simulink library "carnot"  (R2018b)
settings: Solver=VariableStepAuto  StartTime=0.0  StopTime=10.0  RelTol=1e-3
undefined symbols (not defined in the file or in its folder): A, A_earth, acol, Acol, ActPower1, ActPower2, ActPower3, Ad, Ad0, Ar, Au, Au0, Azimuth_Angle, B, Bd, Bd0, Br, Bu, Bu0, C, c1, c2, c3, c33, c4, c5, c6, CarnotCallbacks_Density, CarnotCallbacks_Enthalpy, CarnotCallbacks_Enthalpy2Temperature, CarnotCallbacks_Entropy, CarnotCallbacks_Evaporation_Enthalpy, CarnotCallbacks_GlobalMessageLevel, CarnotCallbacks_Grashof, CarnotCallbacks_Heat_Capacity, CarnotCallbacks_Kinematic_Viscosity, CarnotCallbacks_PMV_PPD, CarnotCallbacks_Prandtl, CarnotCallbacks_Saturation_Property, CarnotCallbacks_Saturation_Temperature, CarnotCallbacks_Saturation_Value_Water, CarnotCallbacks_Specific_Volume, CarnotCallbacks_Thermal_Conductivity, CarnotCallbacks_Vapour_Content, CarnotCallbacks_Vapour_Pressure, Cd, Cdl, Cr, Cu, Davies, Dd, DE_TRY2010_04_averageYear, delta_grd, density, DiameterLastPiece, dl, DPConstant, DPLinear, DPQuadratic, Dr ... (+59)
libraries: $bdroot x429, simulink x36, simulink_extras x12
(part 7 of 22)

== system carnot/Control/Thermostat_Proportional ==
  note: u = (Tset - T + Play/2)
  note: y = operationPoint*(1 + 1/(proportianlRange-Play)) * u
  note: Limit output between 0...1
  T : Inport
  Tset : Inport  Port=2
  Backlash : Backlash  BacklashWidth=bl
  Gain1 : Gain  Gain=0.5
  Play : Constant  Value=bl
  Product : Product  Inputs=**/
  Saturation : Saturate  UpperLimit=1  LowerLimit=0
  Sensor : TransferFcn  Denominator=[ts 1]  mask{ts=ts}
      mask prompts: ts "First order hold for temperature sensor in s"
  Sum1 : Sum  Inputs=-++  SaturateOnIntegerOverflow=on  InputSameDT=on  OutDataTypeStr=Inherit: Same as first input
  Sum2 : Sum  Inputs=-+  SaturateOnIntegerOverflow=on  InputSameDT=on  OutDataTypeStr=Inherit: Same as first input
  Sum3 : Sum  Inputs=2  SaturateOnIntegerOverflow=on  InputSameDT=on  OutDataTypeStr=Inherit: Same as first input
  operationPosition : Constant  Value=op
  proportionalRange : Constant  Value=p
  pos : Outport
  wires:
  Sensor/1 -> Sum1/1
  Sum1/1 -> Backlash/1
  Backlash/1 -> Product/2  "u"
  Saturation/1 -> pos/1
  Sum3/1 -> Saturation/1
  T/1 -> Sensor/1
  Tset/1 -> Sum1/2
  Play/1 -> Sum2/1, Gain1/1
  Gain1/1 -> Sum1/3
  operationPosition/1 -> Sum3/1, Product/1
  proportionalRange/1 -> Sum2/2
  Sum2/1 -> Product/3
  Product/1 -> Sum3/2

== system carnot/Control/Window_Control ==
  Tamb : Inport
  Troom : Inport  Port=2
  Clock2 : Clock
  Data Type Conversion : DataTypeConversion
  FromMorning : simulink/Logic and Bit Operations/Compare To Constant  relop=>=  const=starttime  OutDataTypeStr=boolean
  J->kWh7 : Gain  Gain=1/3600  SaturateOnIntegerOverflow=on  OutDataTypeStr=Inherit: Same as input  ParamDataTypeStr=Inherit: Same as input
  Logical Operator : Logic  AllPortsSameDT=off  OutDataTypeStr=boolean
  Logical Operator1 : Logic  Inputs=3  AllPortsSameDT=off  OutDataTypeStr=boolean
  Math Function : Math  Operator=rem  SaturateOnIntegerOverflow=on
  MovingAverage : DiscreteFir  Coefficients=ones(1,floor(timeFIR))*(1/floor(timeFIR))  InitialStates=TaIni  SampleTime=3600  AccumDataTypeStr=Inherit: Same as product output  RndMeth=Nearest
  Product : Product  RndMeth=Zero
  RelayTroom : Relay  OnSwitchValue=Topen  OffSwitchValue=Tclose
  Rounding Function : Rounding
  Subtract : Sum  Inputs=+-
  Tamb_GT_Const : simulink/Logic and Bit Operations/Compare To Constant  relop=>=  const=TaTooCold  OutDataTypeStr=boolean
  TillEvening : simulink/Logic and Bit Operations/Compare To Constant  relop=<  const=stoptime  OutDataTypeStr=boolean
  Troom_GE_Tamb : simulink/Logic and Bit Operations/Compare To Constant  relop=>=  const=TrAboveTa  OutDataTypeStr=boolean
  const1 : Constant  Value=24*3600
  OpenWindow : Outport
  wires:
  Clock2/1 -> Math Function/1
  const1/1 -> Math Function/2
  Math Function/1 -> J->kWh7/1
  J->kWh7/1 -> Rounding Function/1
  Rounding Function/1 -> TillEvening/1, FromMorning/1  "hourOfTheDay"
  TillEvening/1 -> Logical Operator/1
  FromMorning/1 -> Logical Operator/2
  Tamb/1 -> Subtract/2, MovingAverage/1  "Tamb"
  Logical Operator/1 -> Logical Operator1/3  "daytime"
  Troom/1 -> Subtract/1, RelayTroom/1  "Troom"
  Subtract/1 -> Troom_GE_Tamb/1  "Tr-Ta"
  Troom_GE_Tamb/1 -> Logical Operator1/1  "Troom_GE_Tamb"
  Logical Operator1/1 -> Data Type Conversion/1
  Tamb_GT_Const/1 -> Logical Operator1/2  "Tamb_GT_Const"
  Data Type Conversion/1 -> Product/2
  Product/1 -> OpenWindow/1
  RelayTroom/1 -> Product/1  "TroomTooWarm"
  MovingAverage/1 -> Tamb_GT_Const/1  "TambAvg"

== system carnot/Hydraulics/Fan_Const ==
  THB_Air : Inport
  Ctrl : Inport  Port=2
  Pump_Const : $bdroot/Hydraulics/Pump_Const  mdotmax=Vdotmax/3600*density(Tini,p0,2,0)  dia=dia  p0=p0  fluid_id=Air  mix=mix  mix2=0  mix3=0  UA=UA  mcp=mcp  Tini=Tini  e0=e0  e1=e1  e2=e2
  THB : Outport
  FanDat : Outport  Port=2
  wires:
  Pump_Const/2 -> FanDat/1
  Pump_Const/1 -> THB/1
  Ctrl/1 -> Pump_Const/2  "ControlSetpoint"
  THB_Air/1 -> Pump_Const/1

== system carnot/Hydraulics/Flow_Diverter ==
  THB : Inport
  fdiv : Inport  Port=2
  Bus Assignment : BusAssignment  AssignedSignals=ID,MassFlow,DPConstant,DPLinear,DPQuadratic
  Bus Assignment1 : BusAssignment  AssignedSignals=ID,MassFlow,DPConstant,DPLinear,DPQuadratic
  Bus Selector10 : BusSelector  OutputSignals=MassFlow,DPConstant,DPLinear,DPQuadratic  OutputAsBus=on
  Bus Selector : BusSelector  OutputSignals=MassFlow
  Bus Selector4 : BusSelector  OutputSignals=ID
  Dot Product : DotProduct  InputSameDT=on  OutDataTypeStr=Inherit: Inherit via internal rule
  Saturation : Saturate  UpperLimit=1  LowerLimit=0
  Sum : Sum  Inputs=-+  SaturateOnIntegerOverflow=on  InputSameDT=on  OutDataTypeStr=Inherit: Same as first input
  const{,1..2,4..6} (6 alike) : Constant  Value=0
  increase_ID : Subsystem
  THB1 : Outport
  THB2 : Outport  Port=2
  clq : Outport  Port=3
  wires:
  Bus Selector10/1 -> clq/1
  Bus Assignment1/1 -> THB2/1
  Bus Assignment/1 -> THB1/1
  const4/1 -> Bus Assignment/4  "DPConstant"
  const5/1 -> Bus Assignment/5  "DPLinear"
  const6/1 -> Bus Assignment/6  "DPQuadratic"
  increase_ID/1(Out1) -> Bus Assignment1/2, Bus Assignment/2  "ID"
  Bus Selector4/1 -> increase_ID/1(In1)  "<ID>"
  Dot Product/1 -> Bus Assignment/3, Sum/1  "MassFlow"
  fdiv/1 -> Saturation/1
  THB/1 -> Bus Assignment1/1, Bus Selector10/1, Bus Selector4/1, Bus Assignment/1, Bus Selector/1
  const/1 -> Bus Assignment1/4  "DPConstant"
  Bus Selector/1 -> Sum/2, Dot Product/1  "<MassFlow>"
  Sum/1 -> Bus Assignment1/3  "MassFlow"
  Saturation/1 -> Dot Product/2
  const1/1 -> Bus Assignment1/5  "DPLinear"
  const2/1 -> Bus Assignment1/6  "DPQuadratic"

== system carnot/Hydraulics/Flow_Mixer ==
  THB1 : Inport
  THB2 : Inport  Port=2
  clq : Inport  Port=3
  Calculate_fdiv : Subsystem
  Flow_Mixer_basic : $bdroot/Basic/Hydraulics/Flow_Mixer_basic
  THB : Outport
  fdiv : Outport  Port=2
  wires:
  clq/1 -> Flow_Mixer_basic/3
  Calculate_fdiv/1(f_div) -> fdiv/1
  THB1/1 -> Flow_Mixer_basic/1
  THB2/1 -> Flow_Mixer_basic/2
  Flow_Mixer_basic/1 -> THB/1
  Flow_Mixer_basic/2 -> Calculate_fdiv/1(ID_1)
  Flow_Mixer_basic/3 -> Calculate_fdiv/2(ID_2)
  Flow_Mixer_basic/4 -> Calculate_fdiv/3(fdiv)

== system carnot/Hydraulics/Flow_Mixer_Thermostatic ==
  THBhot : Inport
  THBcold : Inport  Port=2
  clq : Inport  Port=3
  Tset : Inport  Port=4
  Bus Selector : BusSelector  OutputSignals=Temperature
  Flow_Mixer_basic : $bdroot/Basic/Hydraulics/Flow_Mixer_basic
  Icontrol_fdiv : Subsystem
  Terminator : Terminator
  THB : Outport
  fdiv : Outport  Port=2
  wires:
  Bus Selector/1 -> Icontrol_fdiv/3(Twarm)  "<Temperature>"
  Flow_Mixer_basic/4 -> Terminator/1
  Tset/1 -> Icontrol_fdiv/4(Tset)
  Flow_Mixer_basic/3 -> Icontrol_fdiv/2(ID_2)
  Flow_Mixer_basic/2 -> Icontrol_fdiv/1(ID_1)
  Flow_Mixer_basic/1 -> Bus Selector/1, THB/1
  clq/1 -> Flow_Mixer_basic/3
  THBcold/1 -> Flow_Mixer_basic/2
  THBhot/1 -> Flow_Mixer_basic/1
  Icontrol_fdiv/1(f_div) -> fdiv/1

== system carnot/Hydraulics/Mixing_Valve ==
  THB_A : Inport
  THB_B : Inport  Port=2
  clq : Inport  Port=3
  Ctrl : Inport  Port=4
  Bus Creator : BusCreator  Inputs=2
  Calculate_fdiv : Subsystem
  Fcn : Fcn  Expr=1-u
  Flow_Mixer_basic : $bdroot/Basic/Hydraulics/Flow_Mixer_basic
  Valve_A : $bdroot/Hydraulics/Valve  vtyp=equal percentage  psi_0=psi_0  kvs=kvs  dt_V=dt_V
  Valve_B : $bdroot/Hydraulics/Valve  vtyp=linear  psi_0=psi_0  kvs=kvs  dt_V=dt_V
  THB_AB : Outport
  fdiv : Outport  Port=2
  pos : Outport  Port=3
  wires:
  Flow_Mixer_basic/4 -> Calculate_fdiv/3(fdiv)
  Flow_Mixer_basic/3 -> Calculate_fdiv/2(ID_2)
  Flow_Mixer_basic/2 -> Calculate_fdiv/1(ID_1)
  Flow_Mixer_basic/1 -> THB_AB/1
  THB_A/1 -> Valve_A/1
  Calculate_fdiv/1(f_div) -> fdiv/1
  clq/1 -> Flow_Mixer_basic/3
  Valve_A/1 -> Flow_Mixer_basic/1
  THB_B/1 -> Valve_B/1
  Ctrl/1 -> Fcn/1, Valve_A/2
  Valve_B/1 -> Flow_Mixer_basic/2
  Bus Creator/1 -> pos/1
  Valve_A/2 -> Bus Creator/1  "pos_A"
  Valve_B/2 -> Bus Creator/2  "pos_B"
  Fcn/1 -> Valve_B/2

== system carnot/Hydraulics/Pipe ==
  Tamb : Inport
  THBin : Inport  Port=2
  Constant : Constant  Value=hgt
  Pipe_basic : $bdroot/Basic/Thermal_Models/Pipe_basic  vol=pi*(dia/2)^2*len  L=len  uloss=uloss  effcond=cond  cwall=cwall  t0=t0  nodes=nodes
  Pressure_Drop_Fix : $bdroot/Basic/Pressure_Drop/Pressure_Drop_Fix  con=0  lin=lin  qua=qua
  Pressure_Drop_changeD : $bdroot/Basic/Pressure_Drop/Pressure_Drop_changeD  dia=dia
  Pressure_Drop_staticHeight : $bdroot/Basic/Pressure_Drop/Pressure_Drop_staticHeight
  THB : Outport
  wires:
  Pipe_basic/2 -> Pressure_Drop_staticHeight/2
  Pipe_basic/1 -> Pressure_Drop_staticHeight/1
  Tamb/1 -> Pipe_basic/1
  THBin/1 -> Pipe_basic/2
  Constant/1 -> Pressure_Drop_staticHeight/3
  Pressure_Drop_staticHeight/1 -> Pressure_Drop_Fix/1
  Pressure_Drop_Fix/1 -> Pressure_Drop_changeD/1
  Pressure_Drop_changeD/1 -> THB/1

== system carnot/Hydraulics/Pipe_BiFlow ==
  note: discharging pipe connection
  note: charging pipe connection
  Tamb : Inport
  THB_1_in : Inport  Port=2
  THB_2_in : Inport  Port=3
  Constant_THB : $bdroot/Source/Simple/Constant_THB  t=20  mdot=0  p=1e5  mID=No Pressure Drop  fluid=Water  mix=0  mix2=0  mix3=0  dia=0.02  hgt=0
  CreateSdat : $bdroot/Basic/Thermal_Models/CreateSdat  volume=volume  stgtype=stgtype
  Pipe_Connection_1 : $bdroot/Storage/Thermal/Storage_Ports/Pipe_Connection  h_in=pipe1inlet  h_out=pipe1outlet  hgt=hgt  dpipe=pipe1dia  dstg=dia  height=-1273.2395  nodes=nodes
  Pipe_Connection_2 : $bdroot/Storage/Thermal/Storage_Ports/Pipe_Connection  h_in=pipe2inlet  h_out=pipe2outlet  hgt=hgt  dpipe=pipe2dia  dstg=dia  height=1273.2395  nodes=nodes
  select_T : Selector  InputPortWidth=nodes  IndexOptions=Index vector (dialog)  Indices=[1 2 3 4 5 6 7 8 9 10]  OutputSizes=1
  sfun_storageTnodes : $bdroot/Basic/Thermal_Models/sfun_storageTnodes  uloss=uwall  ubot=ubot  utop=utop  cond=axcond  volume=volume  dia=dia  standing=standing cylinder  tini=tini  nodes=nodes  nconnect=2  elimthermocline=0  condinvtc=0
  Sdat : Outport
  THB_1_out : Outport  Port=2
  THB_2_out : Outport  Port=3
  wires:
  Constant_THB/1 -> CreateSdat/15, CreateSdat/8, CreateSdat/9, CreateSdat/10, CreateSdat/11, CreateSdat/12, CreateSdat/13, CreateSdat/14
  Pipe_Connection_1/1 -> sfun_storageTnodes/2
  Pipe_Connection_1/2 -> THB_1_out/1, CreateSdat/5  "THBoutPipe1"
  THB_1_in/1 -> Pipe_Connection_1/2, CreateSdat/4  "THBinPipe1"
  CreateSdat/1 -> Sdat/1
  sfun_storageTnodes/2 -> select_T/1, Pipe_Connection_1/1, Pipe_Connection_2/1  "Tnodes"
  select_T/1 -> CreateSdat/3  "Tnodes"
  Tamb/1 -> CreateSdat/1, sfun_storageTnodes/1  "Tamb"
  THB_2_in/1 -> CreateSdat/6, Pipe_Connection_2/2  "THBinPipe2"
  Pipe_Connection_2/1 -> sfun_storageTnodes/3
  Pipe_Connection_2/2 -> THB_2_out/1, CreateSdat/7  "THBoutPipe2"
  sfun_storageTnodes/1 -> CreateSdat/2  "Energy"

== system carnot/Hydraulics/Pipe_Geometry ==
  Tamb : Inport
  THBin : Inport  Port=2
  Constant : Constant  Value=hgt
  Pipe_basic : $bdroot/Basic/Thermal_Models/Pipe_basic  vol=pi*(dia/2)^2*len  L=len  uloss=uloss  effcond=cond  cwall=cwall  t0=t0  nodes=nodes
  Pressure_Drop_PipeTheory : $bdroot/Basic/Pressure_Drop/Pressure_Drop_PipeTheory  dia=dia  len=len  rough=rough  nbend=nbend
  Pressure_Drop_changeD : $bdroot/Basic/Pressure_Drop/Pressure_Drop_changeD  dia=dia
  Pressure_Drop_staticHeight : $bdroot/Basic/Pressure_Drop/Pressure_Drop_staticHeight
  THB : Outport
  wires:
  Pressure_Drop_PipeTheory/1 -> Pressure_Drop_changeD/1
  Pressure_Drop_staticHeight/1 -> Pressure_Drop_PipeTheory/2
  Pressure_Drop_changeD/1 -> THB/1
  Constant/1 -> Pressure_Drop_staticHeight/3
  Pipe_basic/2 -> Pressure_Drop_staticHeight/2
  Pipe_basic/1 -> Pressure_Drop_PipeTheory/1, Pressure_Drop_staticHeight/1
  THBin/1 -> Pipe_basic/2
  Tamb/1 -> Pipe_basic/1

== system carnot/Hydraulics/Pipe_Isolation ==
  Tamb : Inport
  THBin : Inport  Port=2
  Constant : Constant  Value=hgt
  Pipe_basic : $bdroot/Basic/Thermal_Models/Pipe_basic  vol=pi*(dia/2)^2*len  L=len  uloss=uloss  effcond=cond  cwall=cwall  t0=t0  nodes=nodes
  Pressure_Drop_Fix : $bdroot/Basic/Pressure_Drop/Pressure_Drop_Fix  con=0  lin=lin  qua=qua
  Pressure_Drop_changeD : $bdroot/Basic/Pressure_Drop/Pressure_Drop_changeD  dia=dia
  Pressure_Drop_staticHeight : $bdroot/Basic/Pressure_Drop/Pressure_Drop_staticHeight
  THB : Outport
  wires:
  Pipe_basic/2 -> Pressure_Drop_staticHeight/2
  Pipe_basic/1 -> Pressure_Drop_staticHeight/1
  Pressure_Drop_changeD/1 -> THB/1
  Pressure_Drop_Fix/1 -> Pressure_Drop_changeD/1
  Pressure_Drop_staticHeight/1 -> Pressure_Drop_Fix/1
  Constant/1 -> Pressure_Drop_staticHeight/3
  THBin/1 -> Pipe_basic/2
  Tamb/1 -> Pipe_basic/1

== system carnot/Hydraulics/Pump_Additional ==
  note: Correct the negative pressuredrop.
      | Pump head increases the pressure.
  note: Control signal equal to zero switches
      | to negative ID -> no massflow in the
      | pump (and no pressure drop calculations
      | necessary in the components of the
      | hydraulic loop)
  note: Node for thermal losses and to break
      | the algebraic loop in the temperature
  THBin : Inport
  Ctrl : Inport  Port=2
  Abs : Abs
  Bus Assignment : BusAssignment  AssignedSignals=ID,Temperature,Pressure,DiameterLastPiece,DPConstant,DPLinear,DPQuadratic
  Bus Creator : BusCreator  Inputs=5
  Bus Selector1 : BusSelector  OutputSignals=ID
  Bus Selector2 : BusSelector  OutputSignals=MassFlow
  Bus Selector5 : BusSelector  OutputSignals=MassFlow,Pressure
  Demux : Demux  Outputs=3
  ElectricConsumptionPump : $bdroot/Basic/Hydraulics/ElectricConsumptionPump  e0=e0  e1=e1  e2=e2
  Gain{,1..3} (4 alike) : Gain  Gain=-1
  Pressuredrop : $bdroot/Basic/Pressure_Drop/Pressuredrop
  PumpHead : Gain  Gain=a0
  PumpLinear : Constant  Value=a1
  PumpQuadratic : Constant  Value=a2
  Saturation : Saturate  UpperLimit=1  LowerLimit=0
  Switch3 : Switch  Criteria=u2 > Threshold  SaturateOnIntegerOverflow=on  InputSameDT=on
  ThermalNodeTHB : $bdroot/Basic/Thermal_Models/ThermalNodeTHB  UA=UA  mcp=mcp  Tini=Tini
  dia : Constant  Value=dia
  gain1 : Gain  Gain=-1  SaturateOnIntegerOverflow=on  OutDataTypeStr=Inherit: Same as input  ParamDataTypeStr=Inherit: Same as input
  select_clq : Subsystem
  THB : Outport
  Pdat : Outport  Port=2
  wires:
  Saturation/1 -> Switch3/2, PumpHead/1, Bus Creator/4, ElectricConsumptionPump/2  "ControlActual"
  Gain3/1 -> Bus Creator/3  "PumpHead"
  Pressuredrop/1 -> Bus Assignment/4
  Pressuredrop/2 -> Demux/1  "clq_out"
  Pressuredrop/3 -> Gain3/1
  Bus Assignment/1 -> THB/1, Bus Creator/1  "THB"
  Bus Selector2/1 -> ElectricConsumptionPump/1  "<MassFlow>"
  Bus Creator/1 -> Pdat/1  "Pdat"
  ElectricConsumptionPump/1 -> Bus Creator/2  "PowerElectric"
  Ctrl/1 -> Saturation/1, Bus Creator/5  "ControlSetpoint"
  Bus Selector1/1 -> Switch3/1, Abs/1  "<ID>"
  Abs/1 -> gain1/1
  gain1/1 -> Switch3/3
  Switch3/1 -> Bus Assignment/2  "ID"
  Bus Selector5/1 -> Pressuredrop/1  "<MassFlow>"
  dia/1 -> Bus Assignment/5
  THBin/1 -> select_clq/1(THB), Bus Selector2/1, Bus Selector5/1, Bus Selector1/1, ThermalNodeTHB/1, Bus Assignment/1
  PumpHead/1 -> Gain/1
  PumpLinear/1 -> Gain1/1
  PumpQuadratic/1 -> Gain2/1
  Demux/1 -> Bus Assignment/6
  Demux/2 -> Bus Assignment/7
  Demux/3 -> Bus Assignment/8
  ThermalNodeTHB/1 -> Bus Assignment/3
  select_clq/1(clq) -> Pressuredrop/3
  Bus Selector5/2 -> Pressuredrop/2  "<Pressure>"
  Gain/1 -> Pressuredrop/4
  Gain1/1 -> Pressuredrop/5
  Gain2/1 -> Pressuredrop/6

== system carnot/Hydraulics/Pump_Const ==
  THBin : Inport
  Ctrl : Inport  Port=2
  Bus Assignment : BusAssignment  AssignedSignals=Temperature
  Bus Creator : BusCreator  Inputs=5
  Bus Selector : BusSelector  OutputSignals=MassFlow
  ElectricConsumptionPump : $bdroot/Basic/Hydraulics/ElectricConsumptionPump  e0=e0  e1=e1  e2=e2
  PumpHead : Constant  Value=0
  Pump_basic : $bdroot/Hydraulics/Pump_basic  mdotmax=mdotmax  fluid_id=Water  mix=mix  mix2=mix2  mix3=mix3  p0=p0  dia=dia  ID=No Pressure Drop  hgt=0
  Saturation : Saturate  UpperLimit=1  LowerLimit=0
  ThermalNodeTHB : $bdroot/Basic/Thermal_Models/ThermalNodeTHB  UA=UA  mcp=mcp  Tini=Tini
  THB : Outport
  Pdat : Outport  Port=2
  wires:
  ThermalNodeTHB/1 -> Bus Assignment/2
  Saturation/1 -> Pump_basic/2, ElectricConsumptionPump/2, Bus Creator/4  "ControlActual"
  ElectricConsumptionPump/1 -> Bus Creator/2  "PowerElectric"
  Bus Creator/1 -> Pdat/1  "Pdat"
  Bus Assignment/1 -> THB/1, Bus Creator/1  "THB"
  PumpHead/1 -> Bus Creator/3  "PumpHead"
  Pump_basic/1 -> ThermalNodeTHB/1, Bus Selector/1, Bus Assignment/1
  THBin/1 -> Pump_basic/1
  Ctrl/1 -> Bus Creator/5, Saturation/1  "ControlSetpoint"
  Bus Selector/1 -> ElectricConsumptionPump/1  "<MassFlow>"

== system carnot/Hydraulics/Pump_Main ==
  note: Control signal equal to zero switches
      | to negative ID -> no massflow in the
      | pump (and no pressure drop calculations
      | necessary in the components of the
      | hydraulic loop)
  note: solve quadratic equation
      | DPCOnstant + DPLinear * mdot + DPQadraic * mdot^2
      | = a0 + a1 * mdot + a2 * mdot^2
  note: Transfer function to
      | break algebraic loop
      | in the massflow
  note: Node for thermal losses and to break
      | the algebraic loop in the temperature
  THBin : Inport
  Ctrl : Inport  Port=2
  Bus Assignment : BusAssignment  AssignedSignals=ID,Temperature,MassFlow,Pressure
  Bus Creator : BusCreator  Inputs=5
  Bus Selector : BusSelector  OutputSignals=ID,DPConstant,DPLinear,DPQuadratic
  ElectricConsumptionPump : $bdroot/Basic/Hydraulics/ElectricConsumptionPump  e0=e0  e1=e1  e2=e2
  Gain{1..4} (4 alike) : Gain  Gain=-1
  Ground : Ground
  ID : Constant  Value=ID  mask{IDpreset=pressure drop}
      mask prompts: IDpreset "Calculation"
      mask init:
      | ID = IDpreset*10000 + 1;
      mask TypeOptions IDpreset: pressure drop | pressure drop and pressure head
  Mux2 : Mux  Inputs=7
  Pressure : Constant  Value=p0
  Pressuredrop : $bdroot/Basic/Pressure_Drop/Pressuredrop
  PumpHead : Gain  Gain=a0
  PumpLinear : Constant  Value=a1
  PumpQuadratic : Constant  Value=a2
  S-Function : S-Function  FunctionName=pump  SFunctionDeploymentMode=off  EnableBusSupport=off
  Saturation : Saturate  UpperLimit=1  LowerLimit=0
  Switch1 : Switch  Criteria=u2 > Threshold  SaturateOnIntegerOverflow=on  InputSameDT=on
  Switch3 : Switch  Criteria=u2 > Threshold  SaturateOnIntegerOverflow=on  InputSameDT=on
  Terminator : Terminator
  ThermalNodeTHB : $bdroot/Basic/Thermal_Models/ThermalNodeTHB  UA=UA  mcp=mcp  Tini=Tini
  Transfer Fcn : TransferFcn  Denominator=[t1 1]  mask{t1=t1}
      mask prompts: t1 "Time constant of PT1 transfer function for massflow in s"
  basic_THB : $bdroot/Basic/Hydraulics/basic_THB  t=20  mdot=0  p=p0  ID=No Pressure Drop  fluid=Water  mix=mix  mix2=mix2  mix3=mix3  dia=dia  hgt=0
  const5 : Constant  Value=0
  gain1 : Gain  Gain=-1  SaturateOnIntegerOverflow=on  OutDataTypeStr=Inherit: Same as input  ParamDataTypeStr=Inherit: Same as input
  THB : Outport
  Pdat : Outport  Port=2
  wires:
  Gain4/1 -> Bus Creator/3  "PumpHead"
  Gain2/1 -> Pressuredrop/6
  Gain1/1 -> Pressuredrop/5
  Gain3/1 -> Pressuredrop/4
  Saturation/1 -> Bus Creator/4, ElectricConsumptionPump/2, PumpHead/1, Switch3/2  "ControlActual"
  Pressuredrop/2 -> Terminator/1
  Ground/1 -> Pressuredrop/3
  Pressuredrop/1 -> Bus Assignment/5
  Pressure/1 -> Pressuredrop/2
  Bus Selector/4 -> Mux2/4  "<DPQuadratic>"
  Bus Selector/3 -> Mux2/3  "<DPLinear>"
  Bus Selector/2 -> Mux2/2  "<DPConstant>"
  ThermalNodeTHB/1 -> Bus Assignment/3
  Switch3/1 -> Bus Assignment/2
  Bus Assignment/1 -> Bus Creator/1, THB/1  "THB"
  basic_THB/1 -> Bus Assignment/1
  const5/1 -> Switch1/3
  Transfer Fcn/1 -> Switch1/1, Pressuredrop/1
  gain1/1 -> Switch3/3
  ID/1 -> gain1/1, Switch3/1
  Ctrl/1 -> Bus Creator/5, Saturation/1  "ControlSetpoint"
  PumpHead/1 -> Mux2/5, Gain3/1
  PumpQuadratic/1 -> Mux2/7, Gain2/1
  PumpLinear/1 -> Mux2/6, Gain1/1
  S-Function/1 -> Transfer Fcn/1
  Mux2/1 -> S-Function/1
  Switch1/1 -> ElectricConsumptionPump/1, Bus Assignment/4  "MassFlow"
  Bus Selector/1 -> Mux2/1, Switch1/2  "<ID>"
  Pressuredrop/3 -> Gain4/1
  THBin/1 -> ThermalNodeTHB/1, Bus Selector/1
  Bus Creator/1 -> Pdat/1  "Pdat"
  ElectricConsumptionPump/1 -> Bus Creator/2  "PowerElectric"

== system carnot/Hydraulics/Pump_basic ==
  THBin : Inport
  Ctrl : Inport  Port=2
  Bus Assignment : BusAssignment  AssignedSignals=Temperature,MassFlow
  Bus Selector : BusSelector  OutputSignals=Temperature
  IC : InitialCondition  Value=20
  basic_THB : $bdroot/Basic/Hydraulics/basic_THB  t=20  mdot=0  p=p0  ID=No Pressure Drop  fluid=Water  mix=mix  mix2=mix2  mix3=mix3  dia=dia  hgt=hgt
  mdot : Gain  Gain=mdotmax  SaturateOnIntegerOverflow=on  OutDataTypeStr=Inherit: Same as input  ParamDataTypeStr=Inherit: Same as input
  THB : Outport
  wires:
  IC/1 -> Bus Assignment/2  "Temperature"
  mdot/1 -> Bus Assignment/3  "MassFlow"
  Ctrl/1 -> mdot/1
  THBin/1 -> Bus Selector/1
  Bus Selector/1 -> IC/1  "<Temperature>"
  basic_THB/1 -> Bus Assignment/1
  Bus Assignment/1 -> THB/1

== system carnot/Hydraulics/Thermosyphon ==
  note: Transfer function to
      | break algebraic loop
      | in the massflow
  THBin : Inport
  Bus Assignment : BusAssignment  AssignedSignals=Temperature,MassFlow
  Bus Selector1 : BusSelector  OutputSignals=DPConstant,DPLinear,DPQuadratic  OutputAsBus=on
  Bus Selector2 : BusSelector  OutputSignals=ID
  Bus Selector3 : BusSelector  OutputSignals=GeodeticHeight  OutputAsBus=on
  Bus Selector4 : BusSelector  OutputSignals=Temperature  OutputAsBus=on
  Check difference in height : simulink/Model Verification/Check  Static Range  Description=-0.001 <= u <= 0.001  max=0.001  max_included=on  min=-0.001  min_included=on  enabled=on  stopWhenAssertionFail=on  export=off  icon=graphic
      settings: SourceProductName=Simulink  SourceProductBaseCode=SL
  Mux2 : Mux  Inputs=5
  S-Function : S-Function  FunctionName=pump  SFunctionDeploymentMode=off  EnableBusSupport=off
  Switch1 : Switch  Criteria=u2 > Threshold  SaturateOnIntegerOverflow=on  InputSameDT=on
  Transfer Fcn : $bdroot/Hydraulics/Pump_Main/Transfer Fcn  t1=t1
  basic_THB : $bdroot/Basic/Hydraulics/basic_THB  t=20  mdot=0  p=p0  ID=Full Pressure Drop with Static Height  fluid=Water  mix=mix  mix2=mix2  mix3=mix3  dia=dia  hgt=0
  const{1,3..5} (4 alike) : Constant  Value=0
  THB : Outport
  wires:
  Bus Selector3/1 -> Check difference in height/1
  Switch1/1 -> Bus Assignment/3
  THBin/1 -> Bus Selector4/1, Bus Selector3/1, Bus Selector1/1, Bus Selector2/1
  Bus Selector1/1 -> Mux2/2  "clq"
  Bus Assignment/1 -> THB/1  "THB"
  basic_THB/1 -> Bus Assignment/1
  const5/1 -> Switch1/3
  Transfer Fcn/1 -> Switch1/1
  const1/1 -> Mux2/3
  const4/1 -> Mux2/5
  const3/1 -> Mux2/4
  S-Function/1 -> Transfer Fcn/1
  Mux2/1 -> S-Function/1
  Bus Selector2/1 -> Switch1/2, Mux2/1  "<ID>"
  Bus Selector4/1 -> Bus Assignment/2

== system carnot/Hydraulics/Valve ==
  note: The model is adapted from Thamo_6x2
      | Volkmer (FH Biberach), Carnot User Meeting, Darmstadt, 2018
  THBin : Inport
  Ctrl : Inport  Port=2
  Abs : Abs
  Bus Assignment : BusAssignment  AssignedSignals=ID,Pressure,DPConstant,DPLinear,DPQuadratic
  Bus Selector : BusSelector  OutputSignals=ID,MassFlow,Pressure
  Bus Selector1 : BusSelector  OutputSignals=DPConstant,DPLinear,DPQuadratic  OutputAsBus=on
  Constant : Constant  Value=0
  Constant1 : Constant  Value=0
  Demux : Demux  Outputs=3
  Limit_0_1 : Saturate  UpperLimit=1  LowerLimit=0
  Rate Limiter : RateLimiter  RisingSlewLimit=1/dt_V  FallingSlewLimit=-1/dt_V  SampleTimeMode=inherited  mask{dt_V=dt_V}
      mask prompts: dt_V "Valve running time in s"
  Switch1 : Switch  Criteria=u2 > Threshold  SaturateOnIntegerOverflow=on  InputSameDT=on
  Terminator : Terminator
  gain2 : Gain  Gain=-1  SaturateOnIntegerOverflow=on  OutDataTypeStr=Inherit: Same as input  ParamDataTypeStr=Inherit: Same as input
  pressuredrop : $bdroot/Basic/Pressure_Drop/Pressuredrop
  relFlowCoeff2qua : $bdroot/Basic/Pressure_Drop/relFlowCoeff2qua  kvs=kvs
  relFlowCoefficientFunction : Subsystem  mask{vtyp=linear, psi_0=psi_0}
      mask prompts: vtyp "Valve characteristic"; psi_0 "Relative flow coefficient at zero opening"
      mask TypeOptions vtyp: linear | equal percentage
      mask TypeOptions psi_0: EqualPercentageCharacteristic/psi_0 | LinearCharacteristic/psi_0 | defaultLinear/psi_0
      mask Display: disp('rel\nFlow Coeff')
  THB : Outport
  pos : Outport  Port=2
  wires:
  Rate Limiter/1 -> pos/1, relFlowCoefficientFunction/1(h)
  relFlowCoeff2qua/1 -> pressuredrop/6
  Limit_0_1/1 -> Rate Limiter/1
  relFlowCoefficientFunction/1(psi) -> relFlowCoeff2qua/2
  gain2/1 -> Switch1/3
  Bus Selector/1 -> Switch1/1, Abs/1  "<ID>"
  Ctrl/1 -> Limit_0_1/1, Switch1/2
  Bus Selector1/1 -> pressuredrop/3  "clq"
  pressuredrop/1 -> Bus Assignment/3  "p"
  Bus Selector/2 -> pressuredrop/1  "<MassFlow>"
  Switch1/1 -> Bus Assignment/2  "ID"
  Abs/1 -> gain2/1
  Bus Selector/3 -> pressuredrop/2  "<Pressure>"
  pressuredrop/2 -> Demux/1  "clq"
  Constant/1 -> pressuredrop/4
  Constant1/1 -> pressuredrop/5
  pressuredrop/3 -> Terminator/1
  THBin/1 -> Bus Selector/1, relFlowCoeff2qua/1, Bus Selector1/1, Bus Assignment/1
  Bus Assignment/1 -> THB/1
  Demux/1 -> Bus Assignment/4
  Demux/2 -> Bus Assignment/5
  Demux/3 -> Bus Assignment/6

== system carnot/Hydraulics/Valve_Thermostatic ==
  THBin : Inport
  Troom : Inport  Port=2
  Tset : Inport  Port=3
  Thermostat_Proportional : $bdroot/Control/Thermostat_Proportional  op=op  bl=bl  p=p  ts=ts
  Valve : $bdroot/Hydraulics/Valve  vtyp=linear  psi_0=psi_0  kvs=kvs  dt_V=dt_V
  THB : Outport
  pos : Outport  Port=2
  wires:
  Valve/1 -> THB/1
  Troom/1 -> Thermostat_Proportional/1
  Tset/1 -> Thermostat_Proportional/2
  THBin/1 -> Valve/1
  Thermostat_Proportional/1 -> Valve/2  "valvePosition"
  Valve/2 -> pos/1

== system carnot/Hydraulics/Valve_table ==
  THBin : Inport
  Ctrl : Inport  Port=2
  Abs : Abs
  Bus Assignment : BusAssignment  AssignedSignals=ID,Pressure,DPConstant,DPLinear,DPQuadratic
  Bus Selector : BusSelector  OutputSignals=ID,MassFlow,Pressure
  Bus Selector1 : BusSelector  OutputSignals=DPConstant,DPLinear,DPQuadratic  OutputAsBus=on
  Constant : Constant  Value=0
  Constant1 : Constant  Value=0
  Demux : Demux  Outputs=3
  Limit_0_1 : Saturate  UpperLimit=1  LowerLimit=0
  Rate Limiter : RateLimiter  RisingSlewLimit=1/dt_V  FallingSlewLimit=-1/dt_V  SampleTimeMode=inherited  mask{dt_V=dt_V}
      mask prompts: dt_V "Valve running time in s"
  Switch1 : Switch  Criteria=u2 > Threshold  SaturateOnIntegerOverflow=on  InputSameDT=on
  Terminator : Terminator
  gain2 : Gain  Gain=-1  SaturateOnIntegerOverflow=on  OutDataTypeStr=Inherit: Same as input  ParamDataTypeStr=Inherit: Same as input
  h2psi_table : Lookup_n-D  NumberOfTableDimensions=1  BreakpointsForDimension1=h  Table=psi  InternalRulePriority=Speed  RndMeth=Simplest  InputSameDT=on
  pressuredrop : $bdroot/Basic/Pressure_Drop/Pressuredrop
  relFlowCoeff2qua : $bdroot/Basic/Pressure_Drop/relFlowCoeff2qua  kvs=kvs
  THB : Outport
  pos : Outport  Port=2
  wires:
  Demux/3 -> Bus Assignment/6
  Demux/2 -> Bus Assignment/5
  Demux/1 -> Bus Assignment/4
  Bus Assignment/1 -> THB/1
  THBin/1 -> Bus Assignment/1, Bus Selector1/1, relFlowCoeff2qua/1, Bus Selector/1
  pressuredrop/3 -> Terminator/1
  Constant1/1 -> pressuredrop/5
  Constant/1 -> pressuredrop/4
  pressuredrop/2 -> Demux/1  "clq"
  Bus Selector/3 -> pressuredrop/2  "<Pressure>"
  Abs/1 -> gain2/1
  Switch1/1 -> Bus Assignment/2  "ID"
  Bus Selector/2 -> pressuredrop/1  "<MassFlow>"
  pressuredrop/1 -> Bus Assignment/3  "p"
  Bus Selector1/1 -> pressuredrop/3  "clq"
  Ctrl/1 -> Switch1/2, Limit_0_1/1
  Bus Selector/1 -> Abs/1, Switch1/1  "<ID>"
  gain2/1 -> Switch1/3
  h2psi_table/1 -> relFlowCoeff2qua/2
  Limit_0_1/1 -> Rate Limiter/1
  relFlowCoeff2qua/1 -> pressuredrop/6
  Rate Limiter/1 -> h2psi_table/1, pos/1

== system carnot/Load/General ==
  Data_from_File : Subsystem  mask(Data from File){PathName=path_carnot('data'), FileName='ElectricProfile_SHC_IEA_Task44.mat', UserParam=off, DataName=DataName, t_sample=60}
      mask prompts: PathName "Path"; FileName "File"; UserParam "Edit file and path"; DataName "Variable name"; t_sample "Timestep in data"
      mask help:
      | Loads data in a variable in the workspace. A "From Workspace" block in the subsystem uses this variable. The data matrix must contain the time (in s) as a first column. A Unit-Delay with the "Timestep in data" forces the model to a maximum timestep equal to the data timestep.
      | Buttons in the "Picking a file" opens a window to chose a data file:
      | 1) "From selected path"  from the path shown  in the "Selection" frame.
      | 2) "Carnot public data" from the public data folder in Carnot.
      | 3) "Carnot internal data" from the internal data folder in Carnot.
      | You edit "File" and "Path" after activating the checkbox. Enter 'current' as path and the choice will start in the current Matlab directory.
      | You can use the createDatafile.m function to create the files from .csv or other inputs.
      mask init:
      | [ok,DataName,t_sample] = CarnotCallbacks_Data_from_File('LoadData', ...
      |     gcbh, PathName, FileName);
      mask Help: web(fullfile(path_carnot('help'),'Data_from_file.html'),'-helpbrowser')
      mask Callback UserParam: ok = CarnotCallbacks_Data_from_File('UserMaskEnable',gcbh);
      mask DialogControl ParameterGroupVar Prompt: Picking a file
      mask DialogControl Control2 Prompt: From selected path
      mask DialogControl Control2 Callback: ok = CarnotCallbacks_Data_from_File('GetFilename',gcbh, 'selected');
      mask DialogControl Control3 Prompt: Carnot public data
      mask DialogControl Control3 Callback: ok = CarnotCallbacks_Data_from_File('GetFilename',gcbh, 'public');
      mask DialogControl Control4 Prompt: Carnot internal data
      mask DialogControl Control4 Callback: ok = CarnotCallbacks_Data_from_File('GetFilename',gcbh, 'internal');
      mask DialogControl Container3 Prompt: Selection
      mask Display: disp(['Data file:\n', FileName(1:end-4)])
  Load_Data_Button : Subsystem
      settings: OpenFcn=|
      | [filename, pathname, filterindex] = ...
      |    uigetfile( {'*.mat','MAT-files (*.mat)'; ...
      |    '*.*',  'All Files (*.*)'},  'Pick a data file');
      | 
      | if (filterindex > 0)
      |    load(filename)
      | end
      mask Display: disp('double click \nto load data')
  Repeating_Profile : Subsystem  mask(Repeating Profile){period=24*3600, rep_seq_t=[0 6 7 8 9 11 12 13 14 15 17 18 20 21 22]*3600, rep_seq_d=[6 1 1 1 2 1 1 1 1 2 1 2 1 1 2]*3600, rep_seq_y=[4 2 3 2 0 1 3 2 1 0 1 2 4 3 4]*60}
      mask prompts: period "Time period in s"; rep_seq_t "Time values in s"; rep_seq_d "Duration in s"; rep_seq_y "Output values:"
      mask help:
      | Repeating load profile. The period must be larger than the last time value and the time values must be monotonically ingreasing.
      | Duration is a vector with the same number of elements than the time values. Each duration corresponts to one time value.
      | The number of output values must be the same as the number of time values. Each output value corresponds to one time value.
      mask init:
      | if (length(rep_seq_t) ~= length(rep_seq_y)),
      |   error('Length of time vector and output vector must be the same.')
      | elseif (max(rep_seq_t) > period)
      |   error('Time period must be larger than last time value')
      | end
      | 
      | disp_t1 = rep_seq_t'*[1 1];
      | disp_t2 = (rep_seq_t+rep_seq_d)'*[1 1];
      | disp_t = [disp_t1 disp_t2]';
      | disp_t = [0 reshape(disp_t,1,prod(size(disp_t))) period];
      | 
      | disp_y = rep_seq_y'*[1 1 0 0];
      | disp_y = [0 0 reshape(disp_y',1,prod(size(disp_y)))];
      mask Help: web(fullfile(path_carnot('help'),'Repeating_Profile.html'),'-helpbrowser')
      mask Display: plot( disp_t, disp_y )

== system carnot/Load/Hot_Water_Tapping ==
  DHW_Energy_Tapping : Subsystem  mask{mdot_nom=1/60, times=[7     7.1 7.5   8.083 8.25  8.5   8.75  9     9.5   10.5  11.5  11.75 12.75 14.5  15.5  16.5  18    18.25 18.5  19    20.5  21.25 21.5]*3600, energies=[0.105 1.4 0.105 0.105 0.105 0.105 0.105 0.105 0.105 0.105 0.105 0.105 0.315 0.105 0.105 0.105 0.105 0.105 0.105 0.105 0.735 0.105 1.4 ]*36e5, dT_set=[30    30  30    30    30    30    30    30    30    30    30    30    45    30    30    30    30    30    30    30    45    30    30  ], coeffs=[3     6   3     3     3     3     3     3     3     3     3     3     4     3     3     3     3     3     3     3     4     3     6   ]}
      mask prompts: mdot_nom "nominal massflow [kg/s]"; times "vector of start times of taps [s]"; energies "vector of energies of taps [J]"; dT_set "vector of delta set temperatures of taps [K]"; coeffs "vector of coefficients of nominal massflow of taps [-]"
      mask Display: disp('dhw_EN13203')
  EU_Tapping_Cycle : Subsystem  mask(European tapping cycles){eu_tap=M, dTbias=0}
      mask prompts: eu_tap "EU Tapping Cycle Number"; dTbias "Bias on setpoint temperature in K"
      mask help:
      | European tapping cycles developped according to Mandate 324 and used in various standards for energy labelling and eco design of hot water heaters and hot water storage tanks.
      | The check of mean temperature Tm and peak temperature Tp must be done in a post treatment of the simulation data. A bias on the setpoint temperature can be defined. This assures that the tapping temperature is above the (minimum) setpoint given by the tapping cycle.
      mask init:
      | [times, energies, dT_set, mdot] = ...
      |     CarnotCallbacks_EU_Tapping_Cycle(eu_tap, dTbias);
      mask Help: web(fullfile(path_carnot('help'),'EuTappingCycle.html'),'-helpbrowser')
      mask TypeOptions eu_tap: 3XS | XXS | XS | S | M | L | XL | XXL | 3XL | 4XL
      mask Display: disp('EU tapping\n from 3XS\nto 4XL')
  Hot_Water_Datafile : Subsystem  mask(Hot Water Datafile){PathName=path_carnot('data'), FileName='DHWcalc_SFH_200L.mat', Thot=45, Tcold=10, Tamp=3, dshift=-137}
      mask prompts: PathName "Path"; FileName "File"; Thot "Tapping temperature setpoint in °C"; Tcold "Mean temperature in °C"; Tamp "Amplitude of the sine in K"; dshift "Phase shift of the sine in [days]"
      mask help:
      | Hot water consumption with a temperature and massflow profile from a file.
      | The file must contain a matrix with
      | column 1 : time in s
      | column 2 : temperature setpoint for hot water draw-offs in °C
      | Files max be created with the DHW-calc software and the scrpit createDatafile.m.
      | The hot water of the cylinder entering the block is mixed with the cold water to reach the temperature setpoint. The necessary massflow through the cylinder is calculated by this block and set in the outport to the cylinder.
      mask init:
      | [ok,VariableName] = CarnotCallbacks_Data_from_File('LoadData', ...
      |     gcbh, PathName, FileName);
      mask Help: web(fullfile(path_carnot('help'),'HotWaterDatafile.html'),'-helpbrowser')
      mask TypeOptions PathName: Data_from_File/PathName
      mask TypeOptions FileName: Data_from_File/FileName
      mask TypeOptions Thot: T_hot_water/Value
      mask TypeOptions Tcold: T_cold_Water_Sine/T
      mask TypeOptions Tamp: T_cold_Water_Sine/Tamp
      mask TypeOptions dshift: T_cold_Water_Sine/dshift
      mask DialogControl Container4 Prompt: Datafile
      mask DialogControl Control2 Prompt: From selected path
      mask DialogControl Control2 Callback: ok = CarnotCallbacks_Data_from_File('GetFilename',gcbh, 'selected');
      mask DialogControl Control3 Prompt: Carnot public data
      mask DialogControl Control3 Callback: ok = CarnotCallbacks_Data_from_File('GetFilename',gcbh, 'public');
      mask DialogControl Control4 Prompt: Carnot internal data
      mask DialogControl Control4 Callback: ok = CarnotCallbacks_Data_from_File('GetFilename',gcbh, 'internal');
      mask DialogControl Container3 Prompt: Cold water parameters
      mask Display:
      | text(15,120,'T-Mdot-Profile')
      | plot(0,0,140,130,[70,76,78,63,65,70,70,10],[80,78,74,74,78,80,100,100],[23,23,20,10],[43,47,50,50],[10,10,20,28,30,10],[30,20,20,23,30,30],[22,17],[54,54],[20,20],[54,50],[90,90,50,50],[10,-0,-0,10],[63,64],[60,72],[61,62],[38,50],[60,61],[13,27],[90,85,81,76,70,65,59,54,50],[6,4,6,4,6,4,5,3,5],[68,69],[56,68],[68,68],[32,44],[67,67],[13,23],[73,73],[61,71],[73,73],[43,52],[74,73],[21,36],[78,77],[56,67],[79,79],[34,45],[78,77],[9,23],[82,81],[14,26])
  Hot_Water_EU_TappingCycle : Subsystem  mask(European tapping cycles){T_cold_water=10, eu_tap=L, dTbias=0}
      mask prompts: T_cold_water "Temperature of the cold water"; eu_tap "Tapping cycle"; dTbias "Bias on setpoint temperature in K"
      mask help:
      | Domestic hot water consumption defined by the European Tapping Cycles. This block uses the DHW_Energy_Tapping block.
      | The hot water of the cylinder entering the block is mixed with the cold water to reach the temperature setpoint. The necessary massflow through the cylinder is calculated by this block and set in the outport to the cylinder.
      | The check of mean temperature Tm and peak temperature Tp must be done in a post treatment of the simulation data. A bias on the setpoint temperature can be defined. This assures that the tapping temperature is above the (minimum) setpoint given by the tapping cycle.
      mask Help: web(fullfile(path_carnot('help'),'HotWaterEuTappingCycle.html'),'-helpbrowser')
      mask TypeOptions T_cold_water: T_cold_water/Value
      mask TypeOptions eu_tap: EU_Tapping_Cycle/eu_tap
      mask TypeOptions dTbias: EU_Tapping_Cycle/dTbias
      mask Display:
      | text(15,120,'European Tapping Cycle')
      | plot(0,0,140,130,[70,76,78,63,65,70,70,10],[80,78,74,74,78,80,100,100],[23,23,20,10],[43,47,50,50],[10,10,20,28,30,10],[30,20,20,23,30,30],[22,17],[54,54],[20,20],[54,50],[90,90,50,50],[10,-0,-0,10],[63,64],[60,72],[61,62],[38,50],[60,61],[13,27],[90,85,81,76,70,65,59,54,50],[6,4,6,4,6,4,5,3,5],[68,69],[56,68],[68,68],[32,44],[67,67],[13,23],[73,73],[61,71],[73,73],[43,52],[74,73],[21,36],[78,77],[56,67],[79,79],[34,45],[78,77],[9,23],[82,81],[14,26])
  Hot_Water_Energy_Profile : Subsystem  mask(Hot Water Energy Profile){Tcw=10, mdot_nom=0.1, times=[7 12 19]*3600, energies=[4 2 4]*3600000, dT_set=[35 35 35], coeffs=[1 1 1]}
      mask prompts: Tcw "Cold water temperature in °C"; mdot_nom "Nominal massflow [kg/s]"; times "vector of start times [s]"; energies "vector of energies [J]"; dT_set "vector of temperature differences to the cold water [K]"; coeffs "vector of nominal massflow fractions [-]"
      mask help:
      | Domestic hot water consumption defined by an energy profile. This block uses the DHW_Energy_Tapping block.
      | The hot water of the cylinder entering the block is mixed with the cold water to reach the temperature setpoint. The necessary massflow through the cylinder is calculated by this block and set in the outport to the cylinder.
      mask Help: web(fullfile(path_carnot('help'),'HotWaterEnergyProfile.html'),'-helpbrowser')
      mask TypeOptions Tcw: T_cold_water_const/Value
      mask TypeOptions mdot_nom: DHW_Energy_Tapping/mdot_nom
      mask TypeOptions times: DHW_Energy_Tapping/times
      mask TypeOptions energies: DHW_Energy_Tapping/energies
      mask TypeOptions dT_set: DHW_Energy_Tapping/dT_set
      mask TypeOptions coeffs: DHW_Energy_Tapping/coeffs
      mask DialogControl Container3 Prompt: Profile of the water draw-offs
      mask Display:
      | text(15,120,'Energy-Profile')
      | plot(0,0,140,130,[70,76,78,63,65,70,70,10],[80,78,74,74,78,80,100,100],[23,23,20,10],[43,47,50,50],[10,10,20,28,30,10],[30,20,20,23,30,30],[22,17],[54,54],[20,20],[54,50],[90,90,50,50],[10,-0,-0,10],[63,64],[60,72],[61,62],[38,50],[60,61],[13,27],[90,85,81,76,70,65,59,54,50],[6,4,6,4,6,4,5,3,5],[68,69],[56,68],[68,68],[32,44],[67,67],[13,23],[73,73],[61,71],[73,73],[43,52],[74,73],[21,36],[78,77],[56,67],[79,79],[34,45],[78,77],[9,23],[82,81],[14,26])
  Hot_Water_T_Mdot_Profile : Subsystem  VariantControl=Variant3  mask(Hot Water T-Mdot Profile){Thot=45, Tcold=10, Tamp=0, dshift=0, period=24*3600   % one day, rep_seq_t=0  % tapping at 0:00, rep_seq_d=1*3600  % total duration is 2 h, rep_seq_y=1*10/60   % 10 kg/min}
      mask prompts: Thot "Tapping temperature setpoint in °C"; Tcold "Mean temperature in °C"; Tamp "Amplitude of the sine in K"; dshift "Phase shift of the sine in [days]"; period "Period of the sequence in s"; rep_seq_t "Time values tapping start in s"; rep_seq_d "Duration of each tapping in s"; rep_seq_y "Massflow of each tapping in kg/s"
      mask help:
      | Hot water consumption with a temperature and massflow profile.
      | The hot water of the cylinder entering the block is mixed with the cold water to reach the temperature setpoint. The necessary massflow through the cylinder is calculated by this block and set in the outport to the cylinder.
      mask TypeOptions Thot: T_hot_water/Value
      mask TypeOptions Tcold: T_cold_Water_Sine/T
      mask TypeOptions Tamp: T_cold_Water_Sine/Tamp
      mask TypeOptions dshift: T_cold_Water_Sine/dshift
      mask TypeOptions period: mdot_rep_seq/period
      mask TypeOptions rep_seq_t: mdot_rep_seq/rep_seq_t
      mask TypeOptions rep_seq_d: mdot_rep_seq/rep_seq_d
      mask TypeOptions rep_seq_y: mdot_rep_seq/rep_seq_y
      mask DialogControl Container3 Prompt: Cold water parameters
      mask DialogControl Container4 Prompt: Repeating sequence for masslfow
      mask Display:
      | text(15,120,'T-Mdot-Profile')
      | plot(0,0,140,130,[70,76,78,63,65,70,70,10],[80,78,74,74,78,80,100,100],[23,23,20,10],[43,47,50,50],[10,10,20,28,30,10],[30,20,20,23,30,30],[22,17],[54,54],[20,20],[54,50],[90,90,50,50],[10,-0,-0,10],[63,64],[60,72],[61,62],[38,50],[60,61],[13,27],[90,85,81,76,70,65,59,54,50],[6,4,6,4,6,4,5,3,5],[68,69],[56,68],[68,68],[32,44],[67,67],[13,23],[73,73],[61,71],[73,73],[43,52],[74,73],[21,36],[78,77],[56,67],[79,79],[34,45],[78,77],[9,23],[82,81],[14,26])
  T_cold_Water_Location : Subsystem  mask(water tap){loc=Wuerzburg}
      mask prompts: loc "Location"
      mask help:
      | The block models a tap, that produces a constant massflow of a fluid at given times.
      | control = 1 is full massflow, control = 0 is no massflow.
      | The temperature is a sine wave according to:
      |
      | T(out) = T(mean) + T(amplitude) * sin( 2*PI*(SimulationDay + DayPhaseShift) / 365 )
      mask init:
      | switch loc
      |     case 1  % Athens
      |         T = 15;
      |         Tamp = 5;
      |         dshift = -20;
      |         disp('check temperatures for Athens')
      |     case 2  % Barcelona
      |     case 4  % Madrid
      |         T = 13.5;
      |         Tamp = 4.5;
      |         dshift = -19;
      |     case 3  % Lyon
      |         T = 12;
      |         Tamp = 4;
      |         dshift = -80;
      |         disp('check temperatures for Lyon')
      |     case 5  % Stockholm
      |         T = 8.5;
      |         Tamp = 6.4;
      |         dshift = -80;
      |         disp('check temperatures for Stockholm')
      |     case 6  % Wuerzburg
      |         T = 10;
      |         Tamp = 3;
      |         dshift = -137;
      |     case 7  % Zuerich        
      |         T = 9.7;
      |         Tamp = 6.3;
      |         dshift = -60;
      |         disp('check temperatures for Zuerich')
      |     otherwise
      |         T = 10;
      |         Tamp = 3;
      |         dshift = -137;
      | end
      mask Help: eval('man (''water_tap'')')
      mask TypeOptions loc: Athens | Barcelona | Lyon | Madrid | Stockholm | Wuerzburg | Zuerich
      mask Display:
      | str = ['Athens   ';'Barcelona';'Lyon     ';'Madrid   ';'Stockholm';'Wuerzburg';'Zuerich  '];
      | disp(str(loc,:))
  T_cold_Water_Season : Subsystem  mask(water tap){form=sine wave, month1=February, temp1=6, month2=August, temp2=14}
      mask prompts: form "temperature distribution"; month1 "month with min. temp"; temp1 "minimal temperature [°C]"; month2 "month with max. temp"; temp2 "maximal temperature [°C]"
      mask help:
      | The block models a tap, that produces a constant massflow of a fluid at given times.
      | control = 1 is full massflow, control = 0 is no massflow.
      | The temperature of the water varies during the year.
      mask Help: eval('man (''water_tap'')')
      mask TypeOptions form: sine wave | linear
      mask TypeOptions month1: January | February | March | April | May | June | July | August | September | October | November | December
      mask TypeOptions month2: January | February | March | April | May | June | July | August | September | October | November | December
      mask Display: plot(0,-10,115,110,[0,0],[100,0],[100,0],[50,50],[100,70,20,0],[44,70,30,44])
  T_cold_Water_Sine : Subsystem  mask(water tap){T=10, Tamp=3, dshift=-137}
      mask prompts: T "mean temperature [degree centigrade]"; Tamp "amplitude of the sine [k]"; dshift "phase shift of the sine in [days]"
      mask help:
      | The block models a tap, that produces a constant massflow of a fluid at given times.
      | control = 1 is full massflow, control = 0 is no massflow.
      | The temperature is a sine wave according to:
      |
      | T(out) = T(mean) + T(amplitude) * sin( 2*PI*(SimulationDay + DayPhaseShift) / 365 )
      mask Help: eval('man (''water_tap'')')
      mask Display: plot(0,-10,115,110,[0,0],[100,0],[100,0],[50,50],[100,90,80,70,60,50,40,30,20,10,0],[50,38,30,30,38,50,61,69,69,61,50])
  Water_Tap : Subsystem  mask(water tap){dia=0.02, p=2e5}
      mask prompts: dia "diameter at outlet [m]"; p "system pressure [Pa]"
      mask help:
      | The block models a tap, that produces a constant massflow of a fluid at given times.
      | control = 1 is full massflow, control = 0 is no massflow.
      mask init:
      | fluid = 1; %water
      | mix = 0;
      | dia = max(0.001, dia);
      | p = max(p, 0);
      mask Help: eval('man (''water_tap'')')
      mask Display: plot(-10,10,90,90,[44,67,67,45,45,40,40,44],[80,80,72,72,60,60,76,80],[60,45],[90,90],[53,53],[80,90],[24,29,70,75,24],[30,10,10,30,30],[42,42],[32,58],[46,44],[34,54],[38,40],[34,56])
  mdot_annual_profile : Subsystem  mask(Create Massflow Profile){}
      settings: OpenFcn=CarnotCallbacks_mdot_annual_profile('initialize',gcb);
      mask Help: web(fullfile(path_carnot('help'),'mdot_annual_profile.html'),'-helpbrowser')
  mdot_rep_seq : Subsystem  mask(Repeating Tapping Profile){period=24*3600, rep_seq_t=[7 12 19]*3600, rep_seq_d=[0.2 0.1 0.2]*3600, rep_seq_y=[1 1 1]*200/1800}
      mask prompts: period "Time period in s"; rep_seq_t "Time values in s"; rep_seq_d "Duration in s"; rep_seq_y "Output values:"
      mask help:
      | Period must be larger than the last time value.
      | Time values must be monotonically ingreasing. Give one time value for the start of the tapping.
      | Duration is a vector with the same number of elements than the time values. Each duration corresponts to one time value.
      | The number of output values must be the same as the number of time values. Each output value corresponds to one time value.
      mask init: same as carnot/Load/General/Repeating_Profile
      mask Help:
      | Period must be larger than the last time value.
      | Time values must be monotonically ingreasing. Give one time value for the start of the tapping.
      | Duration is a vector with the same number of elements than the time values. Each duration corresponts to one time value.
      | The number of output values must be the same as the number of time values. Each output value corresponds to one time value.
      mask Display: plot( disp_t, disp_y )
